simulink model "ex8"  (R2020a)
settings: Solver=VariableStepDiscrete  StartTime=-pi/4  StopTime=pi/4  RelTol=1e-3
libraries: simulink x1
settings Model: Creator=반달  LastModifiedBy=반달

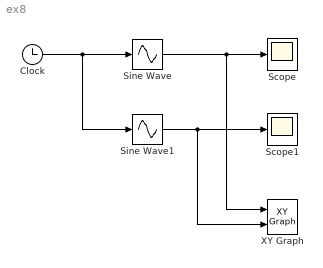
== system ex8 ==
  Clock : Clock
  Scope : Scope
  Scope1 : Scope
  Sine Wave : Sin  TimeSource=Use external signal  Amplitude=0.8  Phase=pi/2  SampleTime=0
  Sine Wave1 : Sin  TimeSource=Use external signal  Amplitude=0.8  SampleTime=0
  XY Graph : simulink/Sinks/XY Graph  xmin=-1  xmax=1  ymin=-1  ymax=1  st=-1
  wires:
  Sine Wave/1 -> Scope/1, XY Graph/1
  Sine Wave1/1 -> XY Graph/2, Scope1/1
  Clock/1 -> Sine Wave/1, Sine Wave1/1
